simulink model "feedbackLin"  (R2021a)
settings: Solver=ode1  StartTime=0.0  StopTime=100  FixedStep=0.05  RelTol=1e-3
undefined symbols (not defined in the file or in its folder): DiscIntNeverNeededParam
settings Model: Creator=laberobotica  LastModifiedBy=gabriel

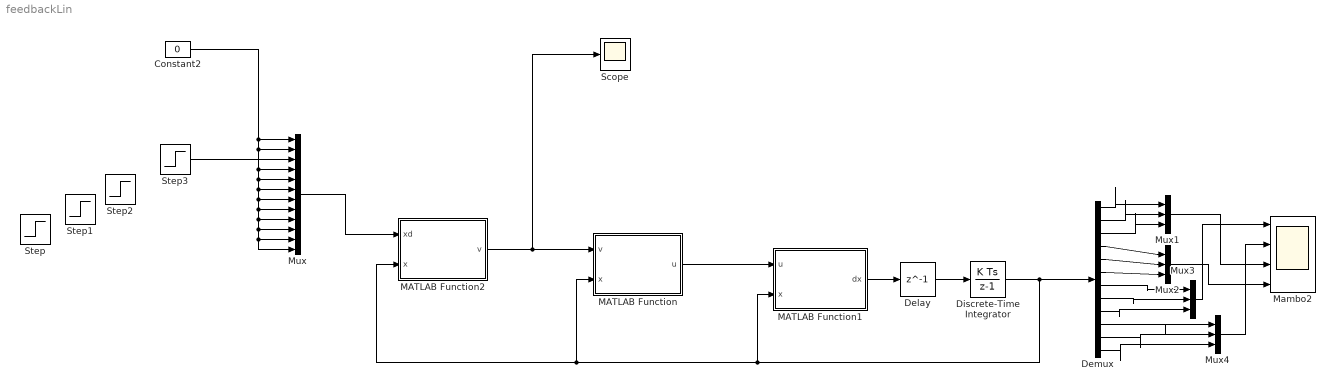
== system feedbackLin ==
  Constant2 : Constant  Value=0
  Delay : Delay  DelayLength=1
  Demux : Demux  Outputs=12
  Discrete-Time Integrator : DiscreteIntegrator  SampleTime=-1  ICPrevOutput=DiscIntNeverNeededParam  ICPrevScaledInput=DiscIntNeverNeededParam
  MATLAB Function : MATLAB Function  TreatAsAtomicUnit=on
  MATLAB Function1 : MATLAB Function  TreatAsAtomicUnit=on
  MATLAB Function2 : MATLAB Function  TreatAsAtomicUnit=on
  Mambo2 : Scope  NumInputPorts=4
  Mux : Mux  Inputs=12
  Mux{1..4} (4 alike) : Mux  Inputs=3
  Scope : Scope
  Step : Step  Time=10  After=pi/4  SampleTime=0
  Step1 : Step  Time=30  After=pi/4  SampleTime=0
  Step2 : Step  Time=50  After=pi/4  SampleTime=0
  Step3 : Step  Before=10  After=10  SampleTime=0
  wires:
  MATLAB Function2/1(v) -> Scope/1, MATLAB Function/1(v)
  MATLAB Function/1(u) -> MATLAB Function1/1(u)
  MATLAB Function1/1(dx) -> Delay/1
  Delay/1 -> Discrete-Time Integrator/1
  Mux/1 -> MATLAB Function2/1(xd)
  Discrete-Time Integrator/1 -> MATLAB Function1/2(x), MATLAB Function/2(x), MATLAB Function2/2(x), Demux/1
  Demux/1 -> Mux1/1
  Demux/2 -> Mux1/2
  Demux/3 -> Mux1/3
  Demux/4 -> Mux2/1
  Demux/5 -> Mux2/2
  Demux/6 -> Mux2/3
  Demux/7 -> Mux3/1
  Demux/8 -> Mux3/2
  Demux/9 -> Mux3/3
  Constant2/1 -> Mux/2, Mux/7, Mux/12, Mux/11, Mux/10, Mux/9, Mux/8, Mux/6, Mux/5, Mux/4, Mux/1
  Demux/10 -> Mux4/1
  Demux/11 -> Mux4/2
  Demux/12 -> Mux4/3
  Mux1/1 -> Mambo2/3
  Mux2/1 -> Mambo2/4
  Mux3/1 -> Mambo2/1
  Mux4/1 -> Mambo2/2
  Step3/1 -> Mux/3

== matlab function feedbackLin/MATLAB Function ==
  data: v input; u output; x input
function u = feedBackLin(v, x)
m = 0.5;
l = 0.2;
Jx = 4.85e-3;
Jy = 4.85e-3;
Jz = 8.81e-3;
g=9.81;
K4 = -8; K3 = -8; K2 = -8;

u = zeros(1,4);


u(1) = m*((v(1)^2)+(v(2)^2)+(g-v(3))^2)^0.5;

u(2) = (Jx/l)*(K2*x(10)-x(11)*x(12)*((Jy-Jz)/Jx))+v(4);
u(3) = (Jy/l)*(K3*x(11)-x(10)*x(12)*((Jz-Jx)/Jy))+v(5);
u(4) = (Jz)*(K4*x(12)-x(10)*x(11)*((Jx-Jy)/Jz))+v(6);
end

== matlab function feedbackLin/MATLAB Function2 ==
  data: xd input; x input; v output
function v = Control(xd,x)

w2 = 0.38; w3 = 0.38; w4 = 0.1;
k1 = 0.1; k2=k1; k3=k2;
v = zeros(1,6);


v(1) = k1*(xd(1) - x(1))+(-xd(1)*x(4));
v(2) = k2*(xd(2) - x(2))+(-xd(2)*x(5));
v(3) = k3*(xd(3) - x(3))+(-xd(3)*x(6));


% controle de orientação
v(4) = w2*(xd(7) - x(7));
v(5) = w3*(xd(8) - x(8));
v(6) = w4*(xd(9) - x(9));


end

== matlab function feedbackLin/MATLAB Function1 ==
  data: u input; dx output; x input
function dx  = DroneModel(u,x)

m = 0.5;
l = 0.2;
Jx = 4.85e-3;
Jy = 4.85e-3;
Jz = 8.81e-3;
g=9.81;

dx = zeros(1,12);

dx(1) = x(4);
dx(2) = x(5);
dx(3) = x(6);

dx(4) = -(cos(x(7)) * sin(x(8)) * cos(x(9)) - sin(x(7))*cos(x(9)))*(u(1)/m);

dx(5) = -(cos(x(7)) * sin(x(8)) * sin(x(9)) + sin(x(7))*cos(x(9)))*(u(1)/m);

dx(6) = g -(cos(x(7)) * cos(x(8)))*(u(1)/m);

dx(7) = x(10);
dx(8) = x(11);
dx(9) = x(12);

dx(10) = x(11)*x(12)*((Jy-Jz)/Jx)+(l/Jx)*u(2);
dx(11) = x(10)*x(12)*((Jz-Jx)/Jy)+(l/Jy)*u(3);
dx(12) = x(10)*x(11)*((Jx-Jy)/Jz)+(1/Jz)*u(4);
end
